simulink model "capitol8prob1"  (R2013a)
settings: Solver=ode45  StartTime=0.0  StopTime=10.0  RelTol=1e-3
undefined symbols (not defined in the file): des, gcbh
settings Model: Creator=user  LastModifiedBy=user

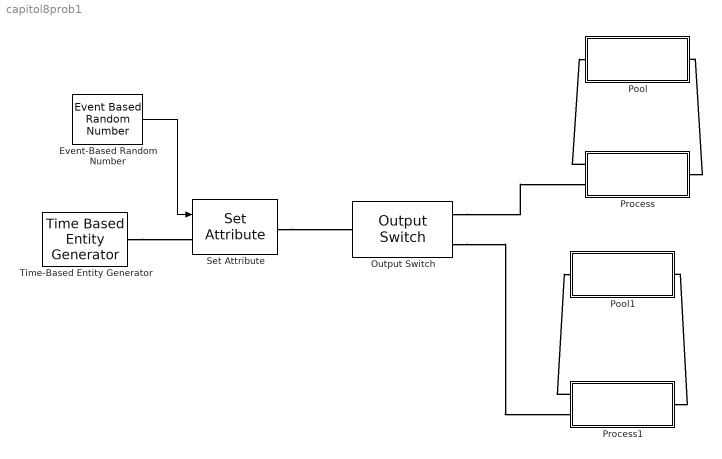
== system capitol8prob1 ==
  Event-Based Random Number : EventBasedRandomNumber  Distribution=Arbitrary discrete  valueVecDisc=[1 2]  probVecDisc=[0.4 0.6]
  Output Switch : OutputSwitch  NumberOutputPorts=2  SwitchingCriterion=From attribute  AttributeName=Type
  Pool : Subsystem
  Pool1 : Subsystem
  Process : Subsystem
  Process1 : Subsystem
  Set Attribute : SetAttribute  AttributeName=Type  AttributeFrom=Signal port  EvaluatedAttributeValue={ []}
  Time-Based Entity Generator : TimeBasedEntityGenerator  Distribution=Uniform  Minimum=0.01  Maximum=0.2
  wires:
  Event-Based Random Number/1 -> Set Attribute/1
  connections:
  Process/RConn1 -- Pool/RConn1
  Time-Based Entity Generator/RConn1 -- Set Attribute/LConn1
  Process/LConn1 -- Pool/LConn1
  Process1/RConn1 -- Pool1/RConn1
  Set Attribute/RConn1 -- Output Switch/LConn1
  Output Switch/RConn2 -- Process1/LConn2
  Output Switch/RConn1 -- Process/LConn2
  Process1/LConn1 -- Pool1/LConn1

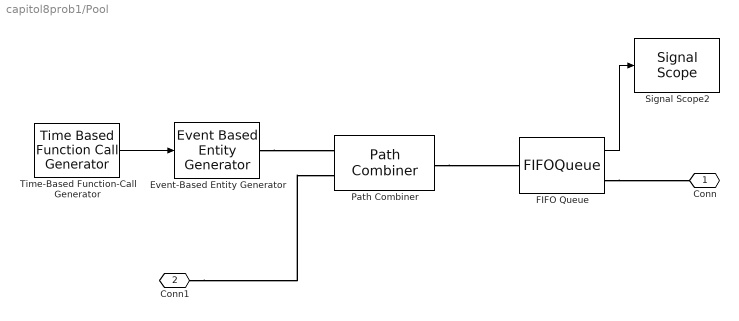
== system capitol8prob1/Pool ==
  Event-Based Entity Generator : EventBasedEntityGenerator  GenerateEntitiesUpon=Function call from port fcn
  FIFO Queue : FIFOQueue  StatNumberInBlock=on
      settings: OutputPortMap=o1
  Path Combiner : PathCombiner  NumberInputPorts=2  InputPortPrecedence=Round robin
  Signal Scope2 : SignalScope  LoadFcn=des.scope.CallbackSupport('seLoadFcn',gcbh)  StartFcn=des.scope.CallbackSupport('seStartFcn',gcbh)  StopFcn=des.scope.CallbackSupport('seStopFcn',gcbh)
      settings: CopyFcn=des.scope.CallbackSupport('seCopyFcn',gcbh)  DeleteFcn=des.scope.CallbackSupport('seDeleteFcn',gcbh)  PreSaveFcn=des.scope.CallbackSupport('sePreSaveFcn',gcbh)  NameChangeFcn=des.scope.CallbackSupport('seNameChangeFcn',gcbh)  OpenFcn=des.scope.CallbackSupport('seOpenFcn',gcbh)
  Time-Based Function-Call Generator : TimeBasedFunctionCallGenerator  EventGenerationMode=Only at simulation start  NumberOfEventsPerPeriod=4
  Conn : PMIOPort  Port=1  Side=Left
  Conn1 : PMIOPort  Port=2  Side=Right
  wires:
  Time-Based Function-Call Generator/1 -> Event-Based Entity Generator/1
  FIFO Queue/1 -> Signal Scope2/1
  connections:
  Path Combiner/RConn1 -- FIFO Queue/LConn1
  Event-Based Entity Generator/RConn1 -- Path Combiner/LConn1
  Conn1/RConn1 -- Path Combiner/LConn2
  FIFO Queue/RConn1 -- Conn/RConn1

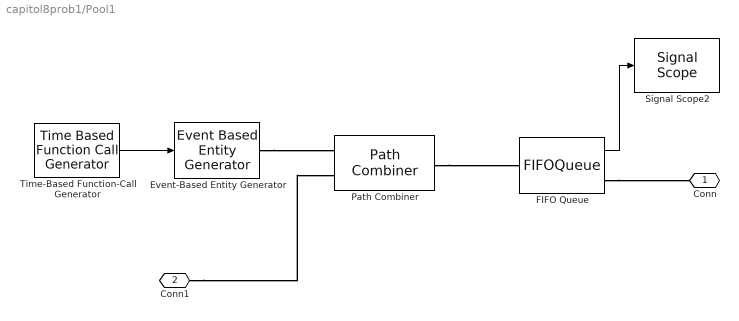
== system capitol8prob1/Pool1 ==
  Event-Based Entity Generator : EventBasedEntityGenerator  GenerateEntitiesUpon=Function call from port fcn
  FIFO Queue : FIFOQueue  StatNumberInBlock=on
      settings: OutputPortMap=o1
  Path Combiner : PathCombiner  NumberInputPorts=2  InputPortPrecedence=Round robin
  Signal Scope2 : SignalScope  LoadFcn=des.scope.CallbackSupport('seLoadFcn',gcbh)  StartFcn=des.scope.CallbackSupport('seStartFcn',gcbh)  StopFcn=des.scope.CallbackSupport('seStopFcn',gcbh)
      settings: CopyFcn=des.scope.CallbackSupport('seCopyFcn',gcbh)  DeleteFcn=des.scope.CallbackSupport('seDeleteFcn',gcbh)  PreSaveFcn=des.scope.CallbackSupport('sePreSaveFcn',gcbh)  NameChangeFcn=des.scope.CallbackSupport('seNameChangeFcn',gcbh)  OpenFcn=des.scope.CallbackSupport('seOpenFcn',gcbh)
  Time-Based Function-Call Generator : TimeBasedFunctionCallGenerator  EventGenerationMode=Only at simulation start  NumberOfEventsPerPeriod=4
  Conn : PMIOPort  Port=1  Side=Left
  Conn1 : PMIOPort  Port=2  Side=Right
  wires:
  Time-Based Function-Call Generator/1 -> Event-Based Entity Generator/1
  FIFO Queue/1 -> Signal Scope2/1
  connections:
  Path Combiner/RConn1 -- FIFO Queue/LConn1
  Event-Based Entity Generator/RConn1 -- Path Combiner/LConn1
  Conn1/RConn1 -- Path Combiner/LConn2
  FIFO Queue/RConn1 -- Conn/RConn1

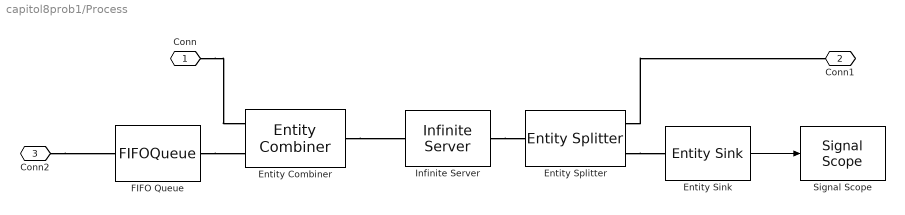
== system capitol8prob1/Process ==
  Entity Combiner : EntityCombiner  NumberInputPorts=2
  Entity Sink : EntitySink  StatNumberArrived=on
  Entity Splitter : EntitySplitter  NumberOutputPorts=2
  FIFO Queue : FIFOQueue  Capacity=4
  Infinite Server : InfiniteServer  ServiceTime=2
  Signal Scope : SignalScope  LoadFcn=des.scope.CallbackSupport('seLoadFcn',gcbh)  StartFcn=des.scope.CallbackSupport('seStartFcn',gcbh)  StopFcn=des.scope.CallbackSupport('seStopFcn',gcbh)
      settings: CopyFcn=des.scope.CallbackSupport('seCopyFcn',gcbh)  DeleteFcn=des.scope.CallbackSupport('seDeleteFcn',gcbh)  PreSaveFcn=des.scope.CallbackSupport('sePreSaveFcn',gcbh)  NameChangeFcn=des.scope.CallbackSupport('seNameChangeFcn',gcbh)  OpenFcn=des.scope.CallbackSupport('seOpenFcn',gcbh)
  Conn : PMIOPort  Port=1  Side=Left
  Conn1 : PMIOPort  Port=2  Side=Right
  Conn2 : PMIOPort  Port=3  Side=Left
  wires:
  Entity Sink/1 -> Signal Scope/1
  connections:
  Entity Splitter/RConn2 -- Entity Sink/LConn1
  Entity Splitter/RConn1 -- Conn1/RConn1
  Infinite Server/RConn1 -- Entity Splitter/LConn1
  Entity Combiner/RConn1 -- Infinite Server/LConn1
  FIFO Queue/RConn1 -- Entity Combiner/LConn2
  Conn/RConn1 -- Entity Combiner/LConn1
  Conn2/RConn1 -- FIFO Queue/LConn1

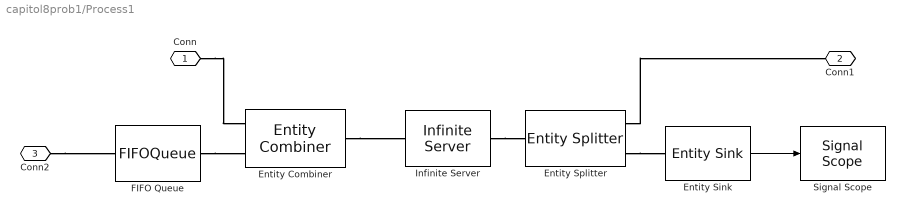
== system capitol8prob1/Process1 ==
  Entity Combiner : EntityCombiner  NumberInputPorts=2
  Entity Sink : EntitySink  StatNumberArrived=on
  Entity Splitter : EntitySplitter  NumberOutputPorts=2
  FIFO Queue : FIFOQueue  Capacity=8
  Infinite Server : InfiniteServer  ServiceTime=3
  Signal Scope : SignalScope  LoadFcn=des.scope.CallbackSupport('seLoadFcn',gcbh)  StartFcn=des.scope.CallbackSupport('seStartFcn',gcbh)  StopFcn=des.scope.CallbackSupport('seStopFcn',gcbh)
      settings: CopyFcn=des.scope.CallbackSupport('seCopyFcn',gcbh)  DeleteFcn=des.scope.CallbackSupport('seDeleteFcn',gcbh)  PreSaveFcn=des.scope.CallbackSupport('sePreSaveFcn',gcbh)  NameChangeFcn=des.scope.CallbackSupport('seNameChangeFcn',gcbh)  OpenFcn=des.scope.CallbackSupport('seOpenFcn',gcbh)
  Conn : PMIOPort  Port=1  Side=Left
  Conn1 : PMIOPort  Port=2  Side=Right
  Conn2 : PMIOPort  Port=3  Side=Left
  wires:
  Entity Sink/1 -> Signal Scope/1
  connections:
  Entity Splitter/RConn2 -- Entity Sink/LConn1
  Entity Splitter/RConn1 -- Conn1/RConn1
  Infinite Server/RConn1 -- Entity Splitter/LConn1
  Entity Combiner/RConn1 -- Infinite Server/LConn1
  FIFO Queue/RConn1 -- Entity Combiner/LConn2
  Conn/RConn1 -- Entity Combiner/LConn1
  Conn2/RConn1 -- FIFO Queue/LConn1
